simulink model "sim_continuo"  (R2015a)
settings: Solver=ode3  StartTime=0.0  StopTime=10  FixedStep=1e-3
values from neighbouring files (symbols this model uses):
  Ki = 2.2902*10^-6    (= 2.2902e-06)    [codex.m]
  Kp = 3.7721*10^-7    (= 3.7721e-07)    [codex.m]
libraries: cstblocks x1
settings Model: Creator=Jose Roldan  LastModifiedBy=Jose Roldan

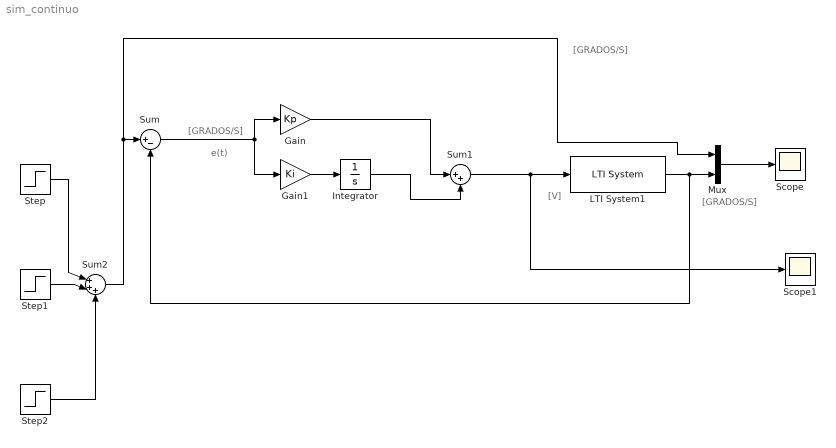
== system sim_continuo ==
  note: e(t)
  note: [GRADOS/S]
  note: [GRADOS/S]
  note: [V]
  note: [GRADOS/S]
  Gain : Gain  Gain=Kp
  Gain1 : Gain  Gain=Ki
  Integrator : Integrator
  LTI System1 : cstblocks/LTI System  sys=G1  IC=[]
  Mux : Mux  Inputs=2
  Scope : Scope
  Scope1 : Scope
  Step : Step  After=3600  SampleTime=0
  Step1 : Step  Time=3  After=6000  SampleTime=0
  Step2 : Step  Time=5  After=5000  SampleTime=0
  Sum : Sum  Inputs=|+-
  Sum1 : Sum  Inputs=|++
  Sum2 : Sum  Inputs=|+++
  wires:
  LTI System1/1 -> Sum/2, Mux/2
  Mux/1 -> Scope/1
  Gain1/1 -> Integrator/1
  Gain/1 -> Sum1/1
  Integrator/1 -> Sum1/2
  Sum1/1 -> LTI System1/1, Scope1/1
  Sum/1 -> Gain1/1, Gain/1
  Step/1 -> Sum2/1
  Step1/1 -> Sum2/2
  Step2/1 -> Sum2/3
  Sum2/1 -> Mux/1, Sum/1
